simulink model "pruebaudp"  (R2025a)
settings: Solver=FixedStepDiscrete  StartTime=0.0  StopTime=inf  FixedStep=0.001  RelTol=1e-3
libraries: etargetslib x1, dspnetwork x1
settings Model: Creator=aero  LastModifiedBy=aero

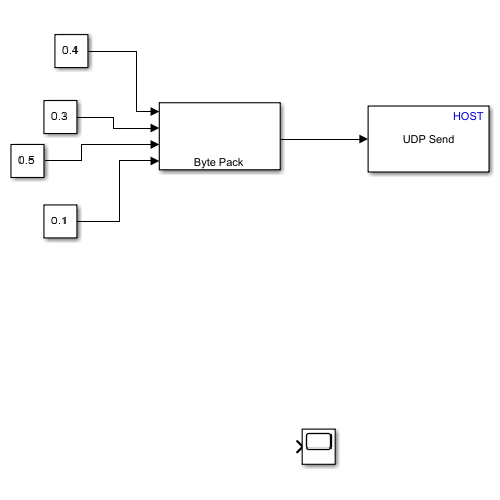
[thumbnail: Simulink's stored preview of the top-level diagram]
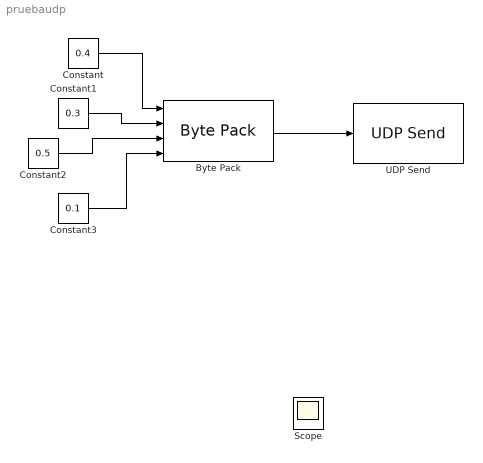
== system pruebaudp ==
  Byte Pack : etargetslib/Byte Pack  datatypes={'double','double','double','double'}  byteAlign=8
  Constant : Constant  Value=0.4
  Constant1 : Constant  Value=0.3
  Constant2 : Constant  Value=0.5
  Constant3 : Constant  Value=0.1
  Scope : Scope
      settings: ActiveDisplayYMinimum=-1.2499999148694405  ActiveDisplayYMaximum=1.2499999903536541
  UDP Send : dspnetwork/UDP Send  remoteURL='127.0.0.1'  remotePort=25000  localURL='0.0.0.0'  localPortSource=Automatically determine  localPort=-1  sendBufferSize=8192  sampletime=-1  blockPlatform=HOST  separateLengthPort=0
      settings: LibrarySourceBlock=embeddedtargetslib/Host Communication/UDP Send
  wires:
  Byte Pack/1 -> UDP Send/1
  Constant3/1 -> Byte Pack/4
  Constant2/1 -> Byte Pack/3
  Constant1/1 -> Byte Pack/2
  Constant/1 -> Byte Pack/1
